simulink model "pid_based_model"  (R2021a)
settings: Solver=VariableStepAuto  StartTime=0.0  StopTime=300  RelTol=1e-3
settings Model: Creator=uddin  LastModifiedBy=uddin
settings SolverCC: ZeroCrossAlgorithm=Adaptive
settings DebuggingCC: IgnoredZcDiagnostic=none

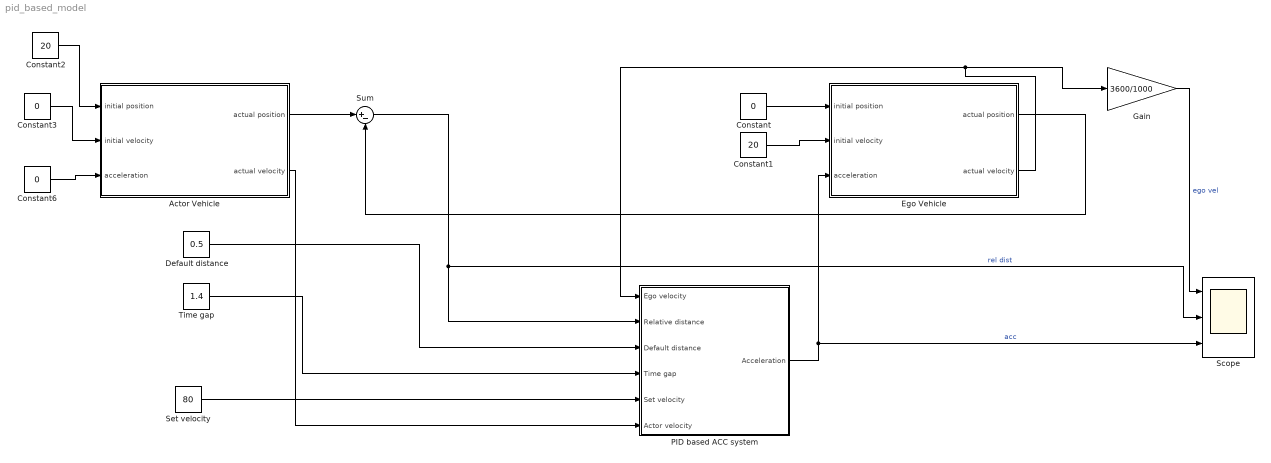
== system pid_based_model ==
  Actor Vehicle : Subsystem
  Constant : Constant  Value=0  SampleTime=.1
  Constant1 : Constant  Value=20  SampleTime=.1
  Constant2 : Constant  Value=20  SampleTime=.1
  Constant3 : Constant  Value=0  SampleTime=.1
  Constant6 : Constant  Value=0  SampleTime=.1
  Default distance : Constant  Value=0.5  SampleTime=.1
  Ego Vehicle : Subsystem
  Gain : Gain  Gain=3600/1000
  PID based ACC system : Subsystem
  Scope : Scope  NumInputPorts=3
  Set velocity : Constant  Value=80  SampleTime=.1
  Sum : Sum  Inputs=|+-
  Time gap : Constant  Value=1.4  SampleTime=.1
  wires:
  Ego Vehicle/1(actual position) -> Sum/2
  Actor Vehicle/1(actual position) -> Sum/1
  Constant/1 -> Ego Vehicle/1(initial position)
  Constant1/1 -> Ego Vehicle/2(initial velocity)
  Constant2/1 -> Actor Vehicle/1(initial position)
  Constant3/1 -> Actor Vehicle/2(initial velocity)
  Ego Vehicle/2(actual velocity) -> PID based ACC system/1(Ego velocity), Gain/1
  Constant6/1 -> Actor Vehicle/3(acceleration)
  Gain/1 -> Scope/1  "ego vel"
  Sum/1 -> PID based ACC system/2(Relative distance), Scope/2  "rel dist"
  Default distance/1 -> PID based ACC system/3(Default distance)
  Time gap/1 -> PID based ACC system/4(Time gap)
  Set velocity/1 -> PID based ACC system/5(Set velocity)
  PID based ACC system/1(Acceleration) -> Ego Vehicle/3(acceleration), Scope/3  "acc"
  Actor Vehicle/2(actual velocity) -> PID based ACC system/6(Actor velocity)

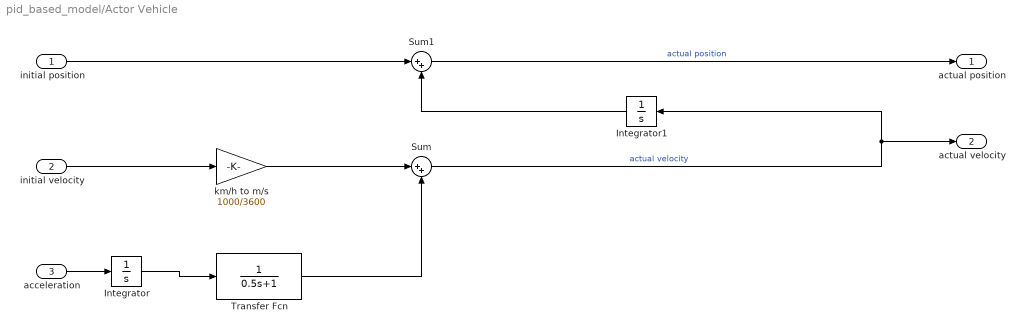
== system pid_based_model/Actor Vehicle ==
  initial position : Inport
  initial velocity : Inport  Port=2
  acceleration : Inport  Port=3
  Integrator : Integrator
  Integrator1 : Integrator
  Sum : Sum  Inputs=|++
  Sum1 : Sum  Inputs=|++
  Transfer Fcn : TransferFcn  Denominator=[0.5 1]
  km/h to m/s : Gain  Gain=1000/3600
  actual position : Outport
  actual velocity : Outport  Port=2
  wires:
  km/h to m/s/1 -> Sum/1
  initial velocity/1 -> km/h to m/s/1
  Transfer Fcn/1 -> Sum/2
  Integrator/1 -> Transfer Fcn/1
  Integrator1/1 -> Sum1/2
  initial position/1 -> Sum1/1
  acceleration/1 -> Integrator/1
  Sum/1 -> Integrator1/1, actual velocity/1  "actual velocity"
  Sum1/1 -> actual position/1  "actual position"

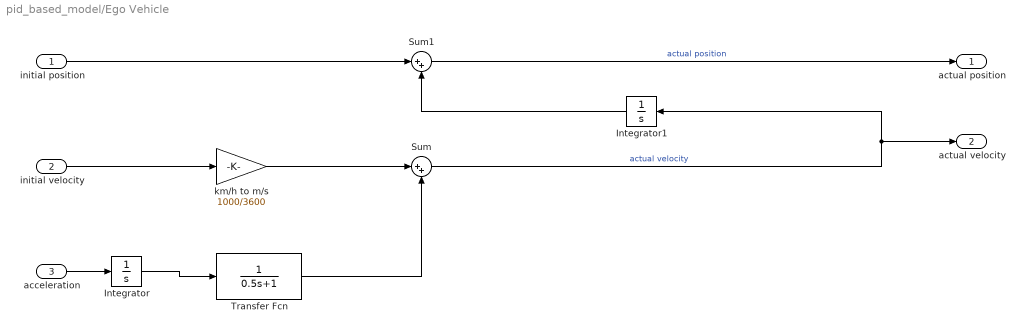
== system pid_based_model/Ego Vehicle ==
  initial position : Inport
  initial velocity : Inport  Port=2
  acceleration : Inport  Port=3
  Integrator : Integrator
  Integrator1 : Integrator
  Sum : Sum  Inputs=|++
  Sum1 : Sum  Inputs=|++
  Transfer Fcn : TransferFcn  Denominator=[0.5 1]
  km/h to m/s : Gain  Gain=1000/3600
  actual position : Outport
  actual velocity : Outport  Port=2
  wires:
  Sum1/1 -> actual position/1  "actual position"
  Sum/1 -> actual velocity/1, Integrator1/1  "actual velocity"
  acceleration/1 -> Integrator/1
  initial position/1 -> Sum1/1
  Integrator1/1 -> Sum1/2
  Integrator/1 -> Transfer Fcn/1
  Transfer Fcn/1 -> Sum/2
  initial velocity/1 -> km/h to m/s/1
  km/h to m/s/1 -> Sum/1

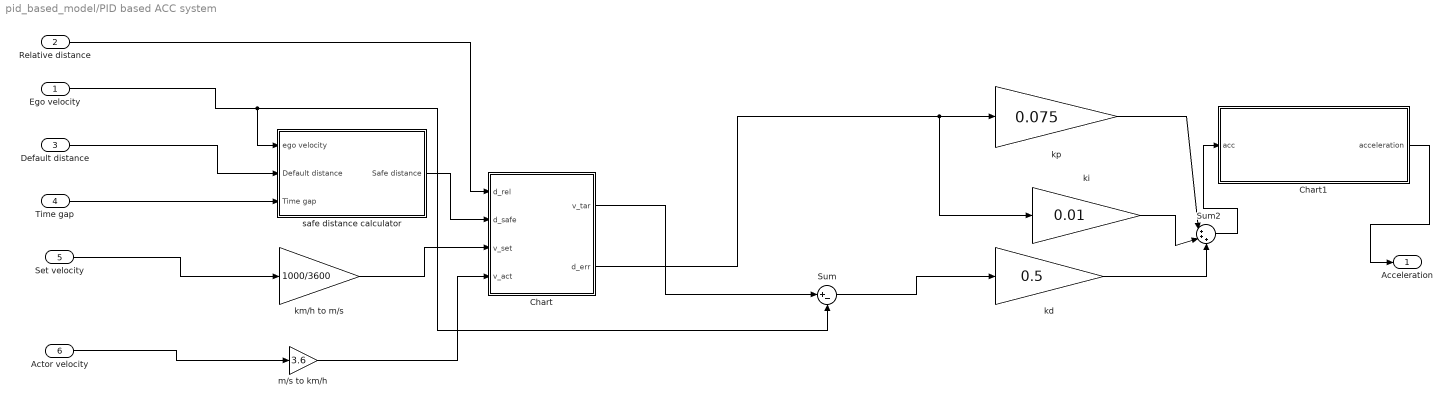
== system pid_based_model/PID based ACC system ==
  Ego velocity : Inport
  Relative distance : Inport  Port=2
  Default distance : Inport  Port=3
  Time gap : Inport  Port=4
  Set velocity : Inport  Port=5
  Actor velocity : Inport  Port=6
  Chart : Stateflow chart  TreatAsAtomicUnit=on
  Chart1 : Stateflow chart  TreatAsAtomicUnit=on
  Sum : Sum  Inputs=|+-
  Sum2 : Sum  Inputs=|+++
  kd : Gain  Gain=0.5
  ki : Gain  Gain=0.01
  km/h to m/s : Gain  Gain=1000/3600
  kp : Gain  Gain=0.075
  m/s to km/h : Gain  Gain=3.6
  safe distance calculator : Subsystem
  Acceleration : Outport
  wires:
  Default distance/1 -> safe distance calculator/2(Default distance)
  Set velocity/1 -> km/h to m/s/1
  Time gap/1 -> safe distance calculator/3(Time gap)
  Ego velocity/1 -> safe distance calculator/1(ego velocity), Sum/2
  kd/1 -> Sum2/3
  ki/1 -> Sum2/2
  kp/1 -> Sum2/1
  Relative distance/1 -> Chart/1(d_rel)
  safe distance calculator/1(Safe distance) -> Chart/2(d_safe)
  km/h to m/s/1 -> Chart/3(v_set)
  Sum2/1 -> Chart1/1(acc)
  Chart1/1(acceleration) -> Acceleration/1
  Sum/1 -> kd/1
  Chart/1(v_tar) -> Sum/1
  Chart/2(d_err) -> ki/1, kp/1
  Actor velocity/1 -> m/s to km/h/1
  m/s to km/h/1 -> Chart/4(v_act)

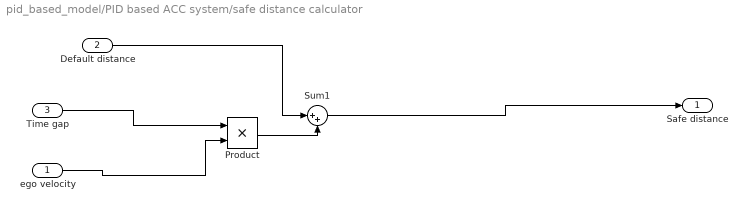
== system pid_based_model/PID based ACC system/safe distance calculator ==
  ego velocity : Inport
  Default distance : Inport  Port=2
  Time gap : Inport  Port=3
  Product : Product
  Sum1 : Sum  Inputs=|++
  Safe distance : Outport
  wires:
  Product/1 -> Sum1/2
  Sum1/1 -> Safe distance/1
  Time gap/1 -> Product/1
  Default distance/1 -> Sum1/1
  ego velocity/1 -> Product/2

== stateflow chart pid_based_model/PID based ACC system/Chart1 ==
  (default) -> (junction 11)
  (junction 11) -> (junction 12) [order 1] : [acc>=3]
  (junction 11) -> (junction 13) [order 2]
  (junction 12) -> (junction 17) : {acceleration=3;}
  (junction 13) -> (junction 14) [order 1] : [acc<=-2]
  (junction 13) -> (junction 15) [order 2] : {acceleration=acc;}
  (junction 14) -> (junction 16) : {acceleration=-2;}
  (junction 16) -> (junction 15)
  (junction 17) -> (junction 16)
  (junction 15) -> (junction 18)
  data: acc input; acceleration output

== stateflow chart pid_based_model/PID based ACC system/Chart ==
  (default) -> (junction 7)
  (junction 7) -> (junction 8) [order 1] : [d_rel>d_safe]
  (junction 7) -> (junction 9) [order 2] : {v_tar=v_act;d_err=d_rel-d_safe;}
  (junction 8) -> (junction 10) : {v_tar=v_set;}
  (junction 10) -> (junction 9)
  (junction 9) -> (junction 11)
  data: d_rel input; d_safe input; v_set input; v_act input; v_tar output; d_err output
